simulink model "Bruss_IO"  (Simulink 8.6)
settings: Solver=ode3  StartTime=0.0  StopTime=10.0  FixedStep=0.2  RelTol=1e-3
libraries: simulink x1
settings Model: Creator=Yi  LastModifiedBy=potok
settings OptimizationCC: DefaultParameterBehavior=Inlined  OptimizeModelRefInitCode=on  LifeSpan=1
settings DebuggingCC: FcnCallInpInsideContextMsg=EnableAllAsWarning
settings RTWCC: SystemTargetFile=ert.tlc  TemplateMakefile=ert_default_tmf  Description=Embedded Coder  Toolchain=GNU gcc/g++ v4.4.x | gmake (64-bit Linux)  TargetLang=C++
settings ERTTargetCC: MultiwordLength=2048  GenerateSampleERTMain=on  MultiInstanceERTCode=on  CodeInterfacePackaging=C++ class  SupportContinuousTime=on  InlinedParameterPlacement=NonHierarchical  RootIOFormat=Structure reference  ERTCustomFileTemplate=example_file_process.tlc  ConvertIfToSwitch=off  SuppressUnreachableDefaultCases=off
settings CPPComponent: GenerateDestructor=on  GenerateExternalIOAccessMethods=None  ParameterMemberVisibility=private  InternalMemberVisibility=private  GenerateParameterAccessMethods=None  GenerateInternalMemberAccessMethods=None  UseOperatorNewForModelRefRegistration=off

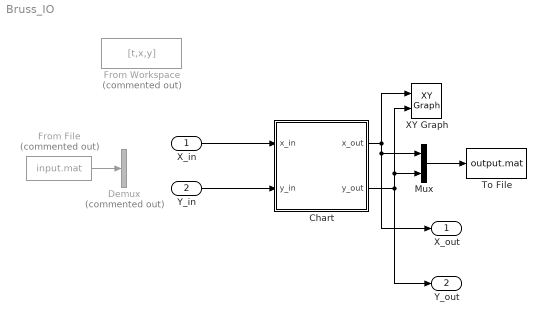
== system Bruss_IO ==
  X_in : Inport
  Y_in : Inport  Port=2
  Chart : Stateflow chart  TreatAsAtomicUnit=on
  Demux : Demux  Commented=on  Outputs=2
  From Workspace : FromWorkspace  Commented=on  VariableName=[t,x,y]  SampleTime=0
  From File : FromFile  Commented=on  FileName=input.mat  SampleTime=0
  Mux : Mux  Inputs=2
  To File : ToFile  Filename=output.mat
  XY Graph : simulink/Sinks/XY Graph  xmin=0  xmax=5  ymin=0  ymax=5  st=-1
  X_out : Outport
  Y_out : Outport  Port=2
  wires:
  Chart/1(x_out) -> X_out/1, Mux/1, XY Graph/1
  From File/1 -> Demux/1
  Mux/1 -> To File/1
  Chart/2(y_out) -> XY Graph/2, Mux/2, Y_out/1
  X_in/1 -> Chart/1(x_in)
  Y_in/1 -> Chart/2(y_in)

== stateflow chart Chart ==
  settings: updateMethod=CONTINUOUS
  state Brussellator
    du:
    x_dot = 1 + x*x*y - 2.5*x;
    y_dot = 1.5*x - x*x*y;
    x_out = x;
    y_out = y;
  note: @annotation-mode=Brussellator;
      | k=2000.0;
      | gamma=0.0;
  (default) -> Brussellator : {x=x_in, y=y_in}
  data: x local double; y local double; x_out output double; y_out output double; x_in input double; y_in input double
  data x settings: updateMethod=SF_CONTINUOUS_TIME_DATA
  data y settings: updateMethod=SF_CONTINUOUS_TIME_DATA
